simulink model "alphabeta_to_abcde"  (R2015a)
settings: Solver=ode3  StartTime=0.0  StopTime=0.1  FixedStep=0.0000001  RelTol=1e-3
libraries: powerlib_meascontrol x1, powerlib x1
settings Model: Creator=hp  LastModifiedBy=hp

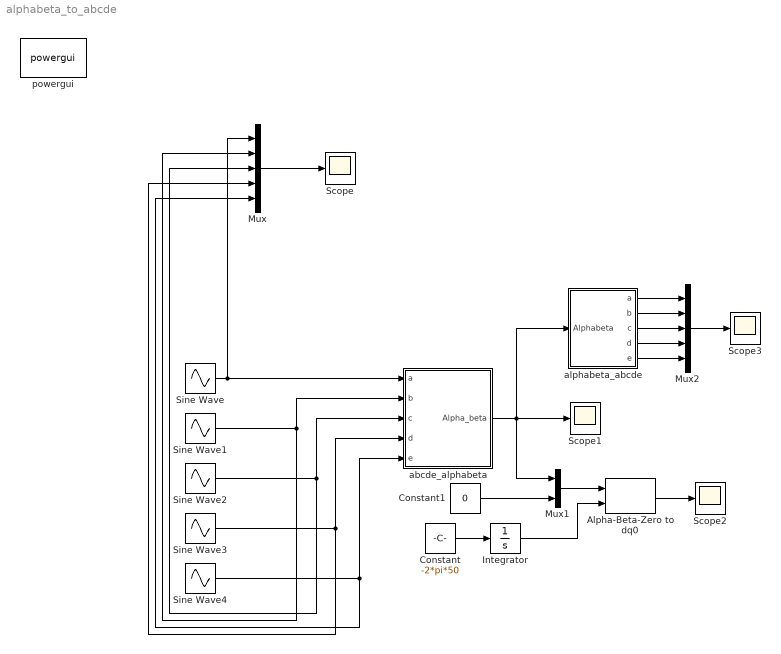
== system alphabeta_to_abcde ==
  Alpha-Beta-Zero to dq0 : powerlib_meascontrol/Transformations/Alpha-Beta-Zero to dq0  Alignment=Aligned with phase A axis
  Constant : Constant  Value=-2*pi*50
  Constant1 : Constant  Value=0
  Integrator : Integrator
  Mux : Mux  Inputs=5
  Mux1 : Mux  Inputs=2
  Mux2 : Mux  Inputs=5
  Scope{,1..3} (4 alike) : Scope
      Scope2 settings: SaveName=ScopeData2
      Scope3 settings: SaveName=ScopeData3
  Sine Wave : Sin  Frequency=2*pi*50  SampleTime=0
  Sine Wave1 : Sin  Frequency=2*pi*50  Phase=2*pi/5  SampleTime=0
  Sine Wave2 : Sin  Frequency=2*pi*50  Phase=4*pi/5  SampleTime=0
  Sine Wave3 : Sin  Frequency=2*pi*50  Phase=6*pi/5  SampleTime=0
  Sine Wave4 : Sin  Frequency=2*pi*50  Phase=8*pi/5  SampleTime=0
  abcde_alphabeta : Subsystem
  alphabeta_abcde : Subsystem
  powergui : powerlib/powergui  Priority=1  SimulationMode=Continuous  SolverType=Tustin/Backward Euler (TBE)  SampleTime=50e-6  frequency=60  SPID=off  DisableSnubberDevices=off  DisableRonSwitches=off  DisableVfSwitches=off  SwTol=0  DisplayEquations=off  Interpol=off  methode=off  Ts=100  FunctionMessages=off  echomessages=off  HookPort=off  EnableUseOfTLC=off  x0status=blocks  frequencyindice=60  Pbase=100e6  ErrMax=1e-4  Iterations=50  UnitsV=kV  UnitsW=MW  buscounter=0  RestoreLinks=warning  ResistiveCurrentMeasurement=off  Frange=[0:2:500]  Ylog=off  Xlog=on  ShowGrid=off  save=off  variable=ZData  structure=0  ZoomFFT=off  StartTime=0.0  cycles=1  DisplayStyle=1  fundamental=60  FreqAxis=off  MaxFrequency=1000  frequencyindicesteady=1  RmsSteady=1  display=off
  wires:
  Mux/1 -> Scope/1
  Sine Wave2/1 -> abcde_alphabeta/3(c), Mux/3
  Sine Wave1/1 -> abcde_alphabeta/2(b), Mux/2
  Sine Wave3/1 -> abcde_alphabeta/4(d), Mux/4
  Sine Wave4/1 -> abcde_alphabeta/5(e), Mux/5
  Sine Wave/1 -> abcde_alphabeta/1(a), Mux/1
  Constant/1 -> Integrator/1
  Mux1/1 -> Alpha-Beta-Zero to dq0/1
  Integrator/1 -> Alpha-Beta-Zero to dq0/2
  Constant1/1 -> Mux1/2
  Alpha-Beta-Zero to dq0/1 -> Scope2/1
  Mux2/1 -> Scope3/1
  abcde_alphabeta/1(Alpha_beta) -> Scope1/1, alphabeta_abcde/1(Alphabeta), Mux1/1
  alphabeta_abcde/1(a) -> Mux2/1
  alphabeta_abcde/2(b) -> Mux2/2
  alphabeta_abcde/3(c) -> Mux2/3
  alphabeta_abcde/4(d) -> Mux2/4
  alphabeta_abcde/5(e) -> Mux2/5

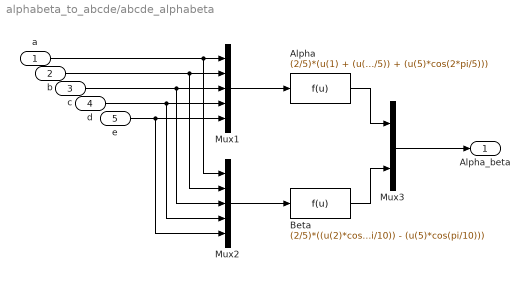
== system alphabeta_to_abcde/abcde_alphabeta ==
  a : Inport
  b : Inport  Port=2
  c : Inport  Port=3
  d : Inport  Port=4
  e : Inport  Port=5
  Alpha : Fcn  Expr=(2/5)*(u(1) + (u(2)*cos(2*pi/5)) + (u(3)*cos(4*pi/5)) + (u(4)*cos(4*pi/5)) + (u(5)*cos(2*pi/5)))
  Beta : Fcn  Expr=(2/5)*((u(2)*cos(pi/10)) + (u(3)*cos(3*pi/10)) - (u(4)*cos(3*pi/10)) - (u(5)*cos(pi/10)))
  Mux1 : Mux  Inputs=5
  Mux2 : Mux  Inputs=5
  Mux3 : Mux  Inputs=2
  Alpha_beta : Outport
  wires:
  Mux1/1 -> Alpha/1
  Beta/1 -> Mux3/2
  Mux2/1 -> Beta/1
  Alpha/1 -> Mux3/1
  Mux3/1 -> Alpha_beta/1
  a/1 -> Mux2/1, Mux1/1
  b/1 -> Mux2/2, Mux1/2
  c/1 -> Mux2/3, Mux1/3
  d/1 -> Mux2/4, Mux1/4
  e/1 -> Mux2/5, Mux1/5

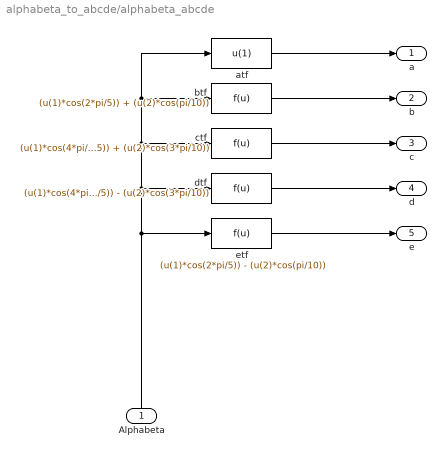
== system alphabeta_to_abcde/alphabeta_abcde ==
  Alphabeta : Inport
  atf : Fcn  Expr=u(1)
  btf : Fcn  Expr=(u(1)*cos(2*pi/5)) + (u(2)*cos(pi/10))
  ctf : Fcn  Expr=(u(1)*cos(4*pi/5)) + (u(2)*cos(3*pi/10))
  dtf : Fcn  Expr=(u(1)*cos(4*pi/5)) - (u(2)*cos(3*pi/10))
  etf : Fcn  Expr=(u(1)*cos(2*pi/5)) - (u(2)*cos(pi/10))
  a : Outport
  b : Outport  Port=2
  c : Outport  Port=3
  d : Outport  Port=4
  e : Outport  Port=5
  wires:
  atf/1 -> a/1
  btf/1 -> b/1
  dtf/1 -> d/1
  etf/1 -> e/1
  ctf/1 -> c/1
  Alphabeta/1 -> etf/1, ctf/1, atf/1, btf/1, dtf/1
